simulink library "csc_mir_miru_lib"  (R2015b)
settings: Solver=ode45  StartTime=0.0  StopTime=10.0  RelTol=1e-3
undefined symbols (not defined in the file or in its folder): sim_time_step_size
libraries: csu_lak_linear_accel_kinematics_lib x4, util_info_lib x1, csu_gyk_gyro_kinematics_lib x1, csu_mhn_miru_hardware_noise_lib x1, csu_rfm_rate_fusion_model_lib x1
settings Model: Creator=escrane  LastModifiedBy=jimkaidy
settings DataIOCC: SaveFormat=Array
settings DebuggingCC: UnderspecifiedInitializationDetection=Classic  MergeDetectMultiDrivingBlocksExec=none  SolverPrmCheckMsg=warning
settings HardwareCC: ProdBitPerPointer=32  ProdLargestAtomicFloat=None  ProdIntDivRoundTo=Undefined  ProdEndianess=Unspecified  ProdWordSize=32  ProdHWDeviceType=32-bit Generic
settings GRTTargetCC: GeneratePreprocessorConditionals=Disable all
settings ConfigComp: CovModelRefEnable=Off  CovSFcnEnable=off

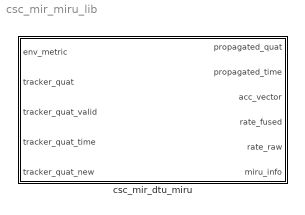
== system csc_mir_miru_lib ==
  csc_mir_dtu_miru : Subsystem

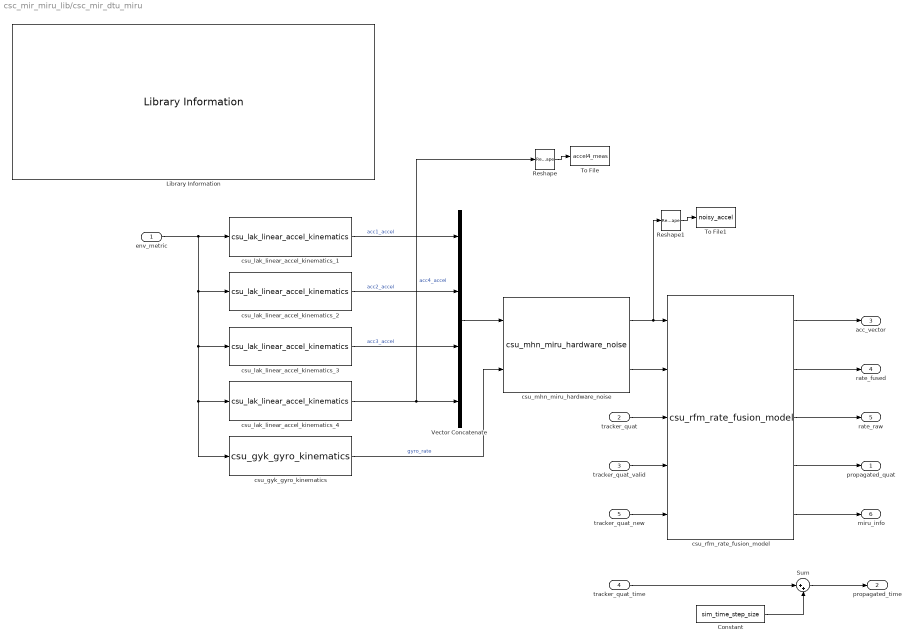
== system csc_mir_miru_lib/csc_mir_dtu_miru ==
  env_metric : Inport
  tracker_quat : Inport  Port=2
  tracker_quat_valid : Inport  Port=3
  tracker_quat_time : Inport  Port=4
  tracker_quat_new : Inport  Port=5
  Constant : Constant  Value=sim_time_step_size  OutDataTypeStr=double
  Library Information : util_info_lib/Library Information  owner='escrane'
  Reshape : Reshape
  Reshape1 : Reshape
  Sum : Sum  Inputs=|++
  To File : ToFile  Filename=accel4_meas  MatrixName=accel4_meas  SaveFormat=Timeseries
  To File1 : ToFile  Filename=noisy_accel  MatrixName=noisy_accel  SaveFormat=Timeseries
  Vector Concatenate : Concatenate  NumInputs=4
  csu_gyk_gyro_kinematics : csu_gyk_gyro_kinematics_lib/csu_gyk_gyro_kinematics
  csu_lak_linear_accel_kinematics_1 : csu_lak_linear_accel_kinematics_lib/csu_lak_linear_accel_kinematics  accel_position=lak_acc1_position  accel_axis_body_frame_1=lak_acc1_direction_1  accel_axis_body_frame_2=lak_acc1_direction_2
  csu_lak_linear_accel_kinematics_2 : csu_lak_linear_accel_kinematics_lib/csu_lak_linear_accel_kinematics  accel_position=lak_acc2_position  accel_axis_body_frame_1=lak_acc2_direction_1  accel_axis_body_frame_2=lak_acc2_direction_2
  csu_lak_linear_accel_kinematics_3 : csu_lak_linear_accel_kinematics_lib/csu_lak_linear_accel_kinematics  accel_position=lak_acc3_position  accel_axis_body_frame_1=lak_acc3_direction_1  accel_axis_body_frame_2=lak_acc3_direction_2
  csu_lak_linear_accel_kinematics_4 : csu_lak_linear_accel_kinematics_lib/csu_lak_linear_accel_kinematics  accel_position=lak_acc4_position  accel_axis_body_frame_1=lak_acc4_direction_1  accel_axis_body_frame_2=lak_acc4_direction_2
  csu_mhn_miru_hardware_noise : csu_mhn_miru_hardware_noise_lib/csu_mhn_miru_hardware_noise
  csu_rfm_rate_fusion_model : csu_rfm_rate_fusion_model_lib/csu_rfm_rate_fusion_model
  propagated_quat : Outport
  propagated_time : Outport  Port=2
  acc_vector : Outport  Port=3
  rate_fused : Outport  Port=4
  rate_raw : Outport  Port=5
  miru_info : Outport  Port=6
  wires:
  csu_rfm_rate_fusion_model/3 -> rate_raw/1
  csu_rfm_rate_fusion_model/2 -> rate_fused/1
  csu_rfm_rate_fusion_model/1 -> acc_vector/1
  csu_mhn_miru_hardware_noise/2 -> csu_rfm_rate_fusion_model/2
  csu_mhn_miru_hardware_noise/1 -> Reshape1/1, csu_rfm_rate_fusion_model/1
  Vector Concatenate/1 -> csu_mhn_miru_hardware_noise/1
  csu_gyk_gyro_kinematics/1 -> csu_mhn_miru_hardware_noise/2  "gyro_rate"
  csu_lak_linear_accel_kinematics_4/1 -> Reshape/1, Vector Concatenate/4  "acc4_accel"
  csu_lak_linear_accel_kinematics_3/1 -> Vector Concatenate/3  "acc3_accel"
  csu_lak_linear_accel_kinematics_2/1 -> Vector Concatenate/2  "acc2_accel"
  csu_lak_linear_accel_kinematics_1/1 -> Vector Concatenate/1  "acc1_accel"
  env_metric/1 -> csu_lak_linear_accel_kinematics_1/1, csu_lak_linear_accel_kinematics_2/1, csu_lak_linear_accel_kinematics_3/1, csu_lak_linear_accel_kinematics_4/1, csu_gyk_gyro_kinematics/1
  csu_rfm_rate_fusion_model/4 -> propagated_quat/1
  csu_rfm_rate_fusion_model/5 -> miru_info/1
  tracker_quat/1 -> csu_rfm_rate_fusion_model/3
  tracker_quat_valid/1 -> csu_rfm_rate_fusion_model/4
  Sum/1 -> propagated_time/1
  tracker_quat_time/1 -> Sum/1
  Constant/1 -> Sum/2
  tracker_quat_new/1 -> csu_rfm_rate_fusion_model/5
  Reshape/1 -> To File/1
  Reshape1/1 -> To File1/1
